simulink model "Lab2_Simulink_Design_Part3_NoPlant"  (R2020a)
settings: Solver=VariableStepAuto  StartTime=0.0  StopTime=10.0  RelTol=1e-3
settings Model: Creator=mati1  LastModifiedBy=mati1

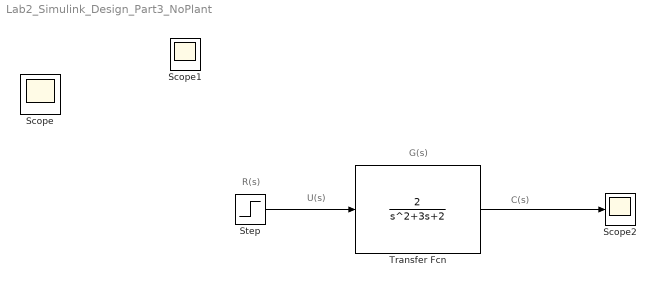
== system Lab2_Simulink_Design_Part3_NoPlant ==
  note: R(s)
  note: U(s)
  note: C(s)
  note: G(s)
  Scope2 : Scope
  Step : Step  Before=1  SampleTime=0
  Transfer Fcn : TransferFcn  Numerator=[2]  Denominator=[1 3 2]
  Scope : Scope
  Scope1 : Scope
  wires:
  Transfer Fcn/1 -> Scope2/1
  Step/1 -> Transfer Fcn/1
